simulink library "mdot_annual_profile"  (R2018b)
settings: Solver=ode45  StartTime=0.0  StopTime=10.0  RelTol=1e-3  EnableMultiTasking=on
libraries: simulink x4
settings Model: Creator=lena.frank  LastModifiedBy=P41573
settings DataIOCC: LimitDataPoints=on  SaveFormat=Array  SignalLoggingSaveFormat=ModelDataLogs
settings OptimizationCC: ExpressionDepthLimit=2147483647  LifeSpan=inf
settings DebuggingCC: UnderspecifiedInitializationDetection=Classic  MergeDetectMultiDrivingBlocksExec=none  SolverPrmCheckMsg=warning  FcnCallInpInsideContextMsg=warning  StateNameClashWarn=warning  SFUnexpectedBacktrackingDiag=warning  SFNoUnconditionalDefaultTransitionDiag=warning  SFExecutionAtInitializationDiag=none
settings HardwareCC: ProdBitPerPointer=32  ProdBitPerSizeT=32  ProdBitPerPtrDiffT=32  ProdLargestAtomicFloat=None  ProdIntDivRoundTo=Undefined  ProdEndianess=Unspecified  ProdWordSize=32  ProdHWDeviceType=32-bit Generic
settings ModelReferenceCC: PropagateSignalLabelsOutOfModel=off
settings SFSimCC: SimUseLocalCustomCode=off
settings RTWCC: RTWUseLocalCustomCode=off
settings CodeAppCC: StateflowObjectComments=on
settings GRTTargetCC: TargetLangStandard=C89/C90 (ANSI)  GeneratePreprocessorConditionals=Disable all  CombineOutputUpdateFcns=off  GRTInterface=on
settings ConfigComp: CovMetricSettings=dw  CovHtmlReporting=on  CovSaveCumulativeToWorkspaceVar=on  CovSaveSingleToWorkspaceVar=on  CovExternalEMLEnable=off

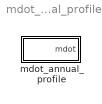
== system mdot_annual_profile ==
  mdot_annual_profile : Subsystem  mask(Create Massflow Profile){}
      settings: OpenFcn=CarnotCallbacks_mdot_annual_profile('initialize',gcb);
      mask Help: web(fullfile(path_carnot('help'),'mdot_annual_profile.html'),'-helpbrowser')

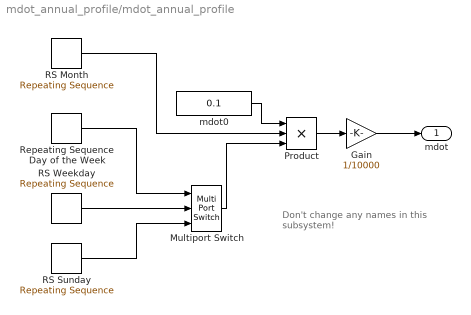
== system mdot_annual_profile/mdot_annual_profile ==
  note: Don't change any names
      | in this subsystem!
  Gain : Gain  Gain=1/10000  SaturateOnIntegerOverflow=on  OutDataTypeStr=Inherit: Same as input  ParamDataTypeStr=Inherit: Same as input
  Multiport Switch : MultiPortSwitch  Inputs=2  SaturateOnIntegerOverflow=on  InputSameDT=on
  Product : Product  Inputs=3  SaturateOnIntegerOverflow=on  InputSameDT=on  OutDataTypeStr=Inherit: Same as first input
  RS Month : simulink/Sources/Repeating Sequence  rep_seq_t=[0 2678399 2678399+1 5097599 5097599+1 7775999 7775999+1 10367999 10367999+1 13046399 13046399+1 15638399 15638399+1 18316799 18316799+1 20995199 20995199+1 23587199 23587199+1 26265599 26265599+1 28857599 28857599+1 31536000]  rep_seq_y=[99 99 97 97 100 100 100 100 103 103 105 105 109 109 112 112 108 108 105 105 101 101 100 100]
  RS Sunday : simulink/Sources/Repeating Sequence  rep_seq_t="100*[0 18 18+1 36 36+1 54 54+1 72 72+1 90 90+1 108 108+1 126 126+1 144 144+1 162 162+1 180 180+1 198 198+1 216 216+1 234 234+1 252 252+1 270 270+1 288 288+1 306 306+1 324 324+1 342 342+1 360 360+1 378 378+1 396 396+1 414 414+1 432 432+1 450 450+1 468 468+1 486 486+1 504 504+1 522 522+1 540 540+1 558 558+1 576 576+1 594 594+1 612 612+1 630 630+1 648 648+1 666 666+1 684 684+1 702 702+1 720 720+1 738 738+1 756 756+1 774 774+1 792 792+1 810 810+1 828 828+1 846 846+1  864]"  rep_seq_y=[0 0 0 0 0.5 0.5 0.5 0.5 0.5 0.5 0.5 0.5 1 1 1 1 1 1 1 1 1 1 1 1 1 1 2 2 2 2 3 3 2 2 2 2 2 2 2 2 3 3 2 2 2 2 2 2 3 3 3 3 3 3 3 3 3 3 2 2 2 2 1 1 1 1 2 2 2 2 3 3 3 3 3 3 3 3 2 2 2 2 2 2 2 2 2 2 1 1 1 1 1 1 1 1]
  RS Weekday : simulink/Sources/Repeating Sequence  rep_seq_t="100*[0 18 18+1 36 36+1 54 54+1 72 72+1 90 90+1 108 108+1 126 126+1 144 144+1 162 162+1 180 180+1 198 198+1 216 216+1 234 234+1 252 252+1 270 270+1 288 288+1 306 306+1 324 324+1 342 342+1 360 360+1 378 378+1 396 396+1 414 414+1 432 432+1 450 450+1 468 468+1 486 486+1 504 504+1 522 522+1 540 540+1 558 558+1 576 576+1 594 594+1 612 612+1 630 630+1 648 648+1 666 666+1 684 684+1 702 702+1 720 720+1 738 738+1 756 756+1 774 774+1 792 792+1 810 810+1 828 828+1 846 846+1  864]"  rep_seq_y=[0.5 0.5 0.5 0.5 0.5 0.5 0.5 0.5 0.5 0.5 0.5 0.5 1 1 1 1 1 1 1 1 2 2 2 2 3 3 3 3 5 5 5 5 5 5 5 5 4 4 4 4 3 3 2 2 2 2 2 2 3 3 3 3 4 4 4 4 3 3 2 2 2 2 1 1 1 1 2 2 2 2 3 3 3 3 3 3 3 3 2 2 2 2 2 2 2 2 2 2 1 1 1 1 1 1 1 1]
  Repeating Sequence Day of the Week : simulink/Sources/Repeating Sequence  rep_seq_t=[0 5*24*3600 5*24*3600+1 7*24*3600]  rep_seq_y=[1 1 2 2]
  mdot0 : Constant  Value=0.1
  mdot : Outport
  wires:
  Repeating Sequence Day of the Week/1 -> Multiport Switch/1
  RS Sunday/1 -> Multiport Switch/3
  Multiport Switch/1 -> Product/3
  mdot0/1 -> Product/1
  Product/1 -> Gain/1
  Gain/1 -> mdot/1
  RS Weekday/1 -> Multiport Switch/2
  RS Month/1 -> Product/2
